simulink library "MCU_MAIN_LIB"  (R2023b)
settings: Solver=VariableStepAuto  StartTime=0.0  StopTime=10.0  RelTol=1e-3
undefined symbols (not defined in the file): BMS_MAIN_LIB, Error_Set_Reset_Deb_100MS, SAMPLE_TIME_100MS, SAMPLE_TIME_100MS_f32, SAMPLE_TIME_10MS
libraries: $bdroot x2, simulink x1
settings Model: Creator=Somashekar M  LastModifiedBy=Somashekar M

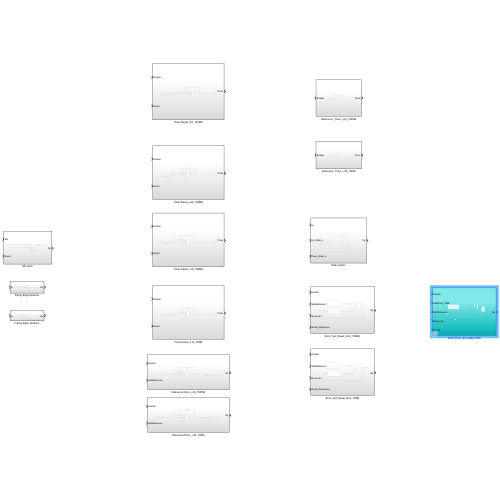
[thumbnail: Simulink's stored preview of the top-level diagram]
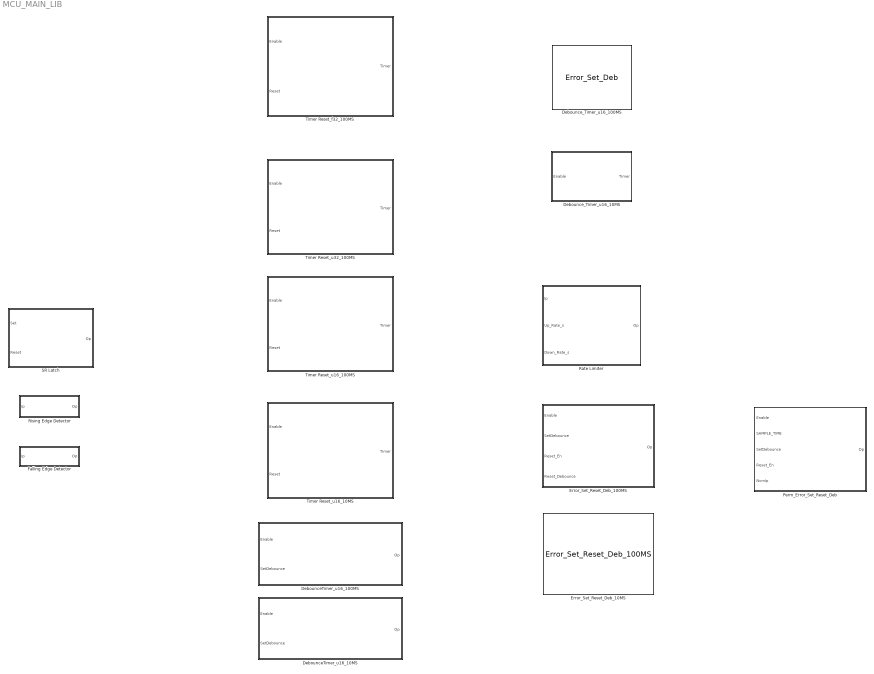
== system MCU_MAIN_LIB ==
  DebounceTimer_u16_100MS : Subsystem
  DebounceTimer_u16_10MS : Subsystem
  Debounce_Timer_u16_100MS : $bdroot/Error_Set_Reset_Deb_100MS/Error_Set_Deb  SystemSampleTime=-1  VariantActivationTime=update diagram  AllowFlexibleInterface=on  Latency=0  AutoFrameSizeCalculation=off
  Debounce_Timer_u16_10MS : Subsystem
  Error_Set_Reset_Deb_100MS : Subsystem
  Error_Set_Reset_Deb_10MS : $bdroot/Error_Set_Reset_Deb_100MS  SystemSampleTime=-1  VariantActivationTime=update diagram  AllowFlexibleInterface=on  Latency=0  AutoFrameSizeCalculation=off
      link override Error_Reset_Deb/Constant7: Value=SAMPLE_TIME_10MS
      link override Error_Set_Deb/Constant7: Value=SAMPLE_TIME_10MS
  Falling Edge Detector : Subsystem
  Perm_Error_Set_Reset_Deb : Subsystem  AncestorBlock=BMS_MAIN_LIB/Error_Set_Reset_Deb_100MS
  Rate Limiter : Subsystem
  Rising Edge Detector : Subsystem
  SR Latch : Subsystem
  Timer Reset_f32_100MS : Subsystem
  Timer Reset_u16_100MS : Subsystem
  Timer Reset_u16_10MS : Subsystem
  Timer Reset_u32_100MS : Subsystem

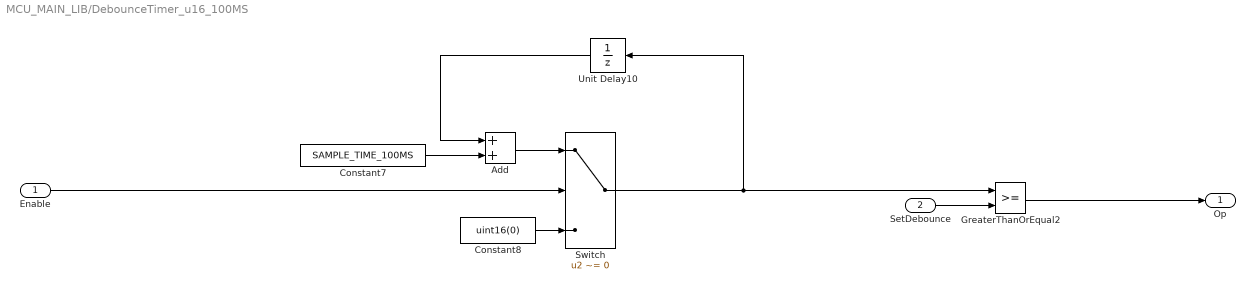
== system MCU_MAIN_LIB/DebounceTimer_u16_100MS ==
  Enable : Inport
  SetDebounce : Inport  Port=2
  Add : Sum
  Constant7 : Constant  Value=SAMPLE_TIME_100MS
  Constant8 : Constant  Value=uint16(0)
  GreaterThanOrEqual2 : RelationalOperator  OutDataTypeStr=boolean  RndMeth=Simplest  InputSameDT=off
  Switch : Switch  Criteria=u2 ~= 0  SaturateOnIntegerOverflow=off  InputSameDT=off
  Unit Delay10 : UnitDelay  SampleTime=-1  HasFrameUpgradeWarning=on
  Op : Outport
  wires:
  Add/1 -> Switch/1
  Constant7/1 -> Add/2
  Enable/1 -> Switch/2
  Unit Delay10/1 -> Add/1
  Constant8/1 -> Switch/3
  Switch/1 -> GreaterThanOrEqual2/1, Unit Delay10/1
  SetDebounce/1 -> GreaterThanOrEqual2/2
  GreaterThanOrEqual2/1 -> Op/1

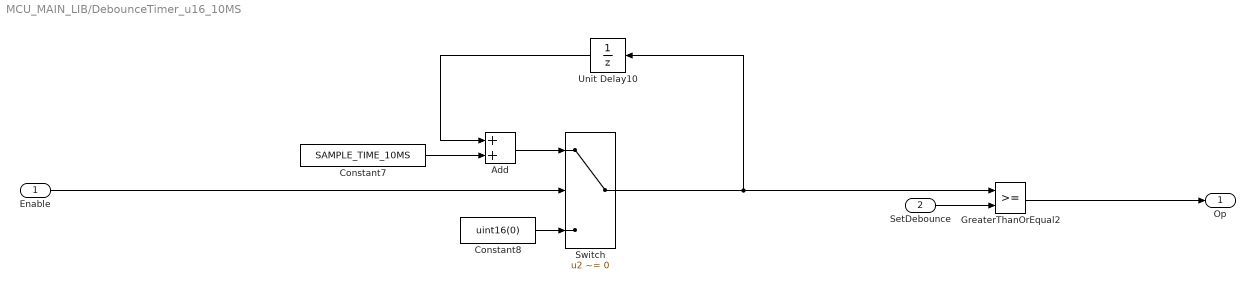
== system MCU_MAIN_LIB/DebounceTimer_u16_10MS ==
  Enable : Inport
  SetDebounce : Inport  Port=2
  Add : Sum
  Constant7 : Constant  Value=SAMPLE_TIME_10MS
  Constant8 : Constant  Value=uint16(0)
  GreaterThanOrEqual2 : RelationalOperator  OutDataTypeStr=boolean  RndMeth=Simplest  InputSameDT=off
  Switch : Switch  Criteria=u2 ~= 0  SaturateOnIntegerOverflow=off  InputSameDT=off
  Unit Delay10 : UnitDelay  SampleTime=-1  HasFrameUpgradeWarning=on
  Op : Outport
  wires:
  GreaterThanOrEqual2/1 -> Op/1
  SetDebounce/1 -> GreaterThanOrEqual2/2
  Switch/1 -> Unit Delay10/1, GreaterThanOrEqual2/1
  Constant8/1 -> Switch/3
  Unit Delay10/1 -> Add/1
  Enable/1 -> Switch/2
  Constant7/1 -> Add/2
  Add/1 -> Switch/1

== system MCU_MAIN_LIB/Debounce_Timer_u16_10MS ==
  Enable : Inport
  Add1 : Sum
  Constant7 : Constant  Value=SAMPLE_TIME_10MS
  Constant8 : Constant  Value=uint16(0)
  Switch2 : Switch  Criteria=u2 ~= 0  SaturateOnIntegerOverflow=off  InputSameDT=off
  Unit Delay10 : UnitDelay  SampleTime=-1  HasFrameUpgradeWarning=on
  Timer : Outport
  wires:
  Switch2/1 -> Timer/1, Unit Delay10/1
  Add1/1 -> Switch2/1
  Constant8/1 -> Switch2/3
  Enable/1 -> Switch2/2
  Unit Delay10/1 -> Add1/1
  Constant7/1 -> Add1/2

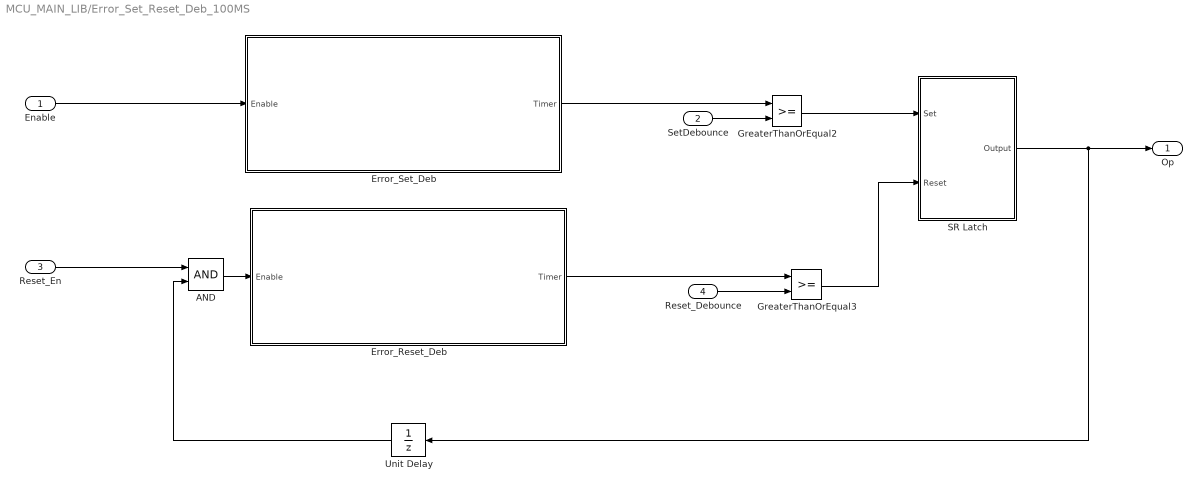
== system MCU_MAIN_LIB/Error_Set_Reset_Deb_100MS ==
  Enable : Inport
  SetDebounce : Inport  Port=2
  Reset_En : Inport  Port=3
  Reset_Debounce : Inport  Port=4
  AND : Logic  AllPortsSameDT=off  OutDataTypeStr=boolean
  Error_Reset_Deb : Subsystem
  Error_Set_Deb : Subsystem
  GreaterThanOrEqual2 : RelationalOperator  OutDataTypeStr=boolean  RndMeth=Simplest  InputSameDT=off
  GreaterThanOrEqual3 : RelationalOperator  OutDataTypeStr=boolean  RndMeth=Simplest  InputSameDT=off
  SR Latch : Subsystem
  Unit Delay : UnitDelay  SampleTime=-1  HasFrameUpgradeWarning=on
  Op : Outport
  wires:
  SetDebounce/1 -> GreaterThanOrEqual2/2
  Reset_Debounce/1 -> GreaterThanOrEqual3/2
  GreaterThanOrEqual3/1 -> SR Latch/2(Reset)
  GreaterThanOrEqual2/1 -> SR Latch/1(Set)
  SR Latch/1(Output) -> Op/1, Unit Delay/1
  AND/1 -> Error_Reset_Deb/1(Enable)
  Error_Set_Deb/1(Timer) -> GreaterThanOrEqual2/1
  Error_Reset_Deb/1(Timer) -> GreaterThanOrEqual3/1
  Reset_En/1 -> AND/1
  Unit Delay/1 -> AND/2
  Enable/1 -> Error_Set_Deb/1(Enable)

== system MCU_MAIN_LIB/Falling Edge Detector ==
  Ip : Inport
  AND : Logic  AllPortsSameDT=off  OutDataTypeStr=boolean
  NOT1 : Logic  Operator=NOT  IconShape=distinctive  AllPortsSameDT=off  OutDataTypeStr=boolean
  Unit Delay : UnitDelay  SampleTime=-1  HasFrameUpgradeWarning=on
  Op : Outport
  wires:
  Unit Delay/1 -> AND/2
  AND/1 -> Op/1
  Ip/1 -> NOT1/1, Unit Delay/1
  NOT1/1 -> AND/1

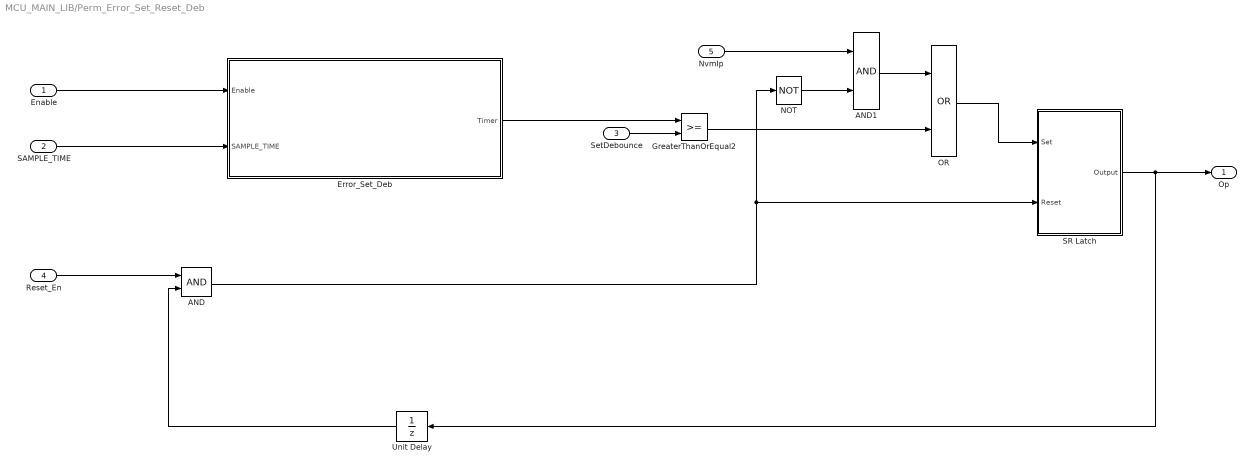
== system MCU_MAIN_LIB/Perm_Error_Set_Reset_Deb ==
  Enable : Inport
  SAMPLE_TIME : Inport  Port=2
  SetDebounce : Inport  Port=3
  Reset_En : Inport  Port=4
  NvmIp : Inport  Port=5
  AND : Logic  AllPortsSameDT=off  OutDataTypeStr=boolean
  AND1 : Logic  AllPortsSameDT=off  OutDataTypeStr=boolean
  Error_Set_Deb : Subsystem
  GreaterThanOrEqual2 : RelationalOperator  OutDataTypeStr=boolean  RndMeth=Simplest  InputSameDT=off
  NOT : Logic  Operator=NOT  IconShape=distinctive  AllPortsSameDT=off  OutDataTypeStr=boolean
  OR : Logic  Operator=OR  AllPortsSameDT=off  OutDataTypeStr=boolean
  SR Latch : Subsystem
  Unit Delay : UnitDelay  SampleTime=-1  HasFrameUpgradeWarning=on
  Op : Outport
  wires:
  Enable/1 -> Error_Set_Deb/1(Enable)
  Unit Delay/1 -> AND/2
  Reset_En/1 -> AND/1
  Error_Set_Deb/1(Timer) -> GreaterThanOrEqual2/1
  SR Latch/1(Output) -> Unit Delay/1, Op/1
  GreaterThanOrEqual2/1 -> OR/2
  AND/1 -> SR Latch/2(Reset), NOT/1
  SetDebounce/1 -> GreaterThanOrEqual2/2
  SAMPLE_TIME/1 -> Error_Set_Deb/2(SAMPLE_TIME)
  OR/1 -> SR Latch/1(Set)
  AND1/1 -> OR/1
  NvmIp/1 -> AND1/1
  NOT/1 -> AND1/2

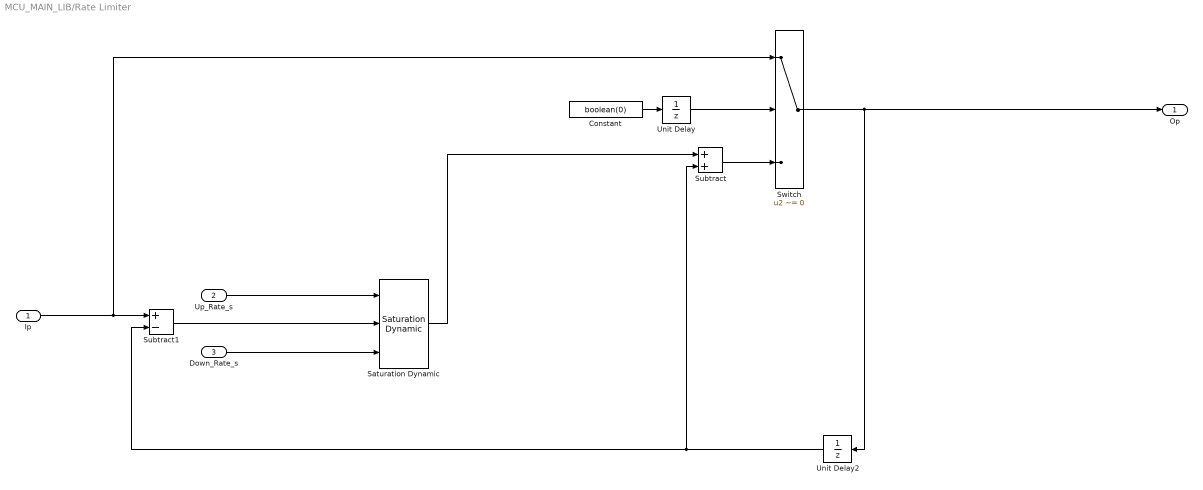
== system MCU_MAIN_LIB/Rate Limiter ==
  Ip : Inport
  Up_Rate_s : Inport  Port=2
  Down_Rate_s : Inport  Port=3
  Constant : Constant  Value=boolean(0)
  Saturation Dynamic : simulink/Discontinuities/Saturation Dynamic  OutMin=[]  OutMax=[]  OutDataTypeStr=Inherit: Same as second input  OutDataType=fixdt(1, 16)  OutScaling=2^-10  DoSatur=off
  Subtract : Sum
  Subtract1 : Sum  Inputs=+-
  Switch : Switch  Criteria=u2 ~= 0  SaturateOnIntegerOverflow=off  InputSameDT=off
  Unit Delay : UnitDelay  InitialCondition=boolean(1)  SampleTime=-1  HasFrameUpgradeWarning=on
  Unit Delay2 : UnitDelay  SampleTime=-1  HasFrameUpgradeWarning=on
  Op : Outport
  wires:
  Subtract/1 -> Switch/3
  Unit Delay/1 -> Switch/2
  Constant/1 -> Unit Delay/1
  Ip/1 -> Switch/1, Subtract1/1
  Down_Rate_s/1 -> Saturation Dynamic/3
  Unit Delay2/1 -> Subtract/2, Subtract1/2
  Subtract1/1 -> Saturation Dynamic/2
  Saturation Dynamic/1 -> Subtract/1
  Switch/1 -> Op/1, Unit Delay2/1
  Up_Rate_s/1 -> Saturation Dynamic/1

== system MCU_MAIN_LIB/Rising Edge Detector ==
  Ip : Inport
  AND : Logic  AllPortsSameDT=off  OutDataTypeStr=boolean
  NOT : Logic  Operator=NOT  IconShape=distinctive  AllPortsSameDT=off  OutDataTypeStr=boolean
  Unit Delay : UnitDelay  SampleTime=-1  HasFrameUpgradeWarning=on
  Op : Outport
  wires:
  Ip/1 -> Unit Delay/1, AND/1
  AND/1 -> Op/1
  NOT/1 -> AND/2
  Unit Delay/1 -> NOT/1

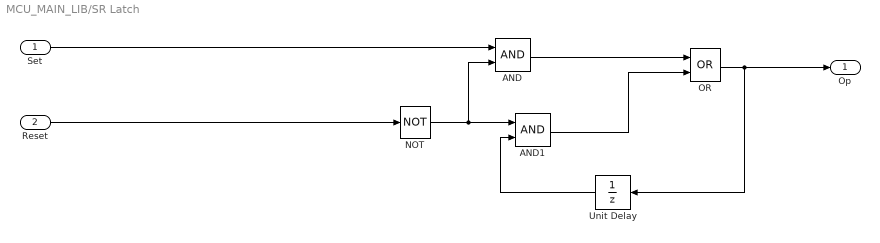
== system MCU_MAIN_LIB/SR Latch ==
  Set : Inport
  Reset : Inport  Port=2
  AND : Logic  AllPortsSameDT=off  OutDataTypeStr=boolean
  AND1 : Logic  AllPortsSameDT=off  OutDataTypeStr=boolean
  NOT : Logic  Operator=NOT  IconShape=distinctive  AllPortsSameDT=off  OutDataTypeStr=boolean
  OR : Logic  Operator=OR  AllPortsSameDT=off  OutDataTypeStr=boolean
  Unit Delay : UnitDelay  SampleTime=-1  HasFrameUpgradeWarning=on
  Op : Outport
  wires:
  Unit Delay/1 -> AND1/2
  Set/1 -> AND/1
  AND1/1 -> OR/2
  NOT/1 -> AND1/1, AND/2
  OR/1 -> Unit Delay/1, Op/1
  AND/1 -> OR/1
  Reset/1 -> NOT/1

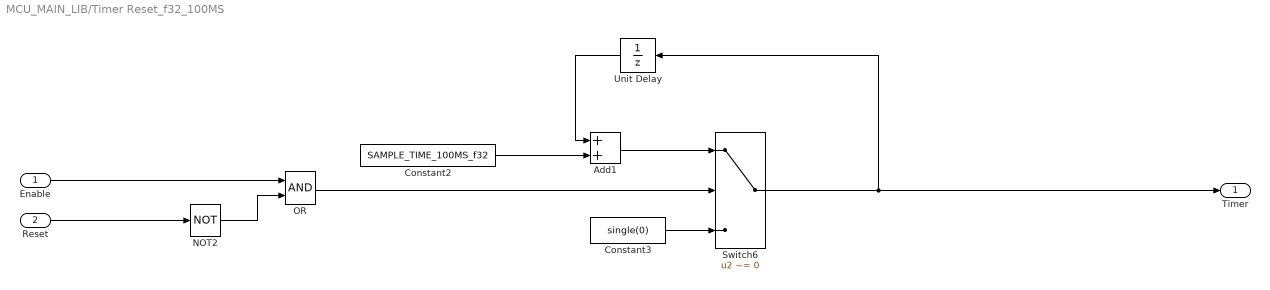
== system MCU_MAIN_LIB/Timer Reset_f32_100MS ==
  Enable : Inport
  Reset : Inport  Port=2
  Add1 : Sum
  Constant2 : Constant  Value=SAMPLE_TIME_100MS_f32  OutDataTypeStr=single
  Constant3 : Constant  Value=single(0)
  NOT2 : Logic  Operator=NOT  IconShape=distinctive  AllPortsSameDT=off  OutDataTypeStr=boolean
  OR : Logic  AllPortsSameDT=off  OutDataTypeStr=boolean
  Switch6 : Switch  Criteria=u2 ~= 0  SaturateOnIntegerOverflow=off  InputSameDT=off
  Unit Delay : UnitDelay  SampleTime=-1  HasFrameUpgradeWarning=on
  Timer : Outport
  wires:
  Enable/1 -> OR/1
  Constant3/1 -> Switch6/3
  Add1/1 -> Switch6/1
  Switch6/1 -> Timer/1, Unit Delay/1
  Reset/1 -> NOT2/1
  NOT2/1 -> OR/2
  OR/1 -> Switch6/2
  Unit Delay/1 -> Add1/1
  Constant2/1 -> Add1/2

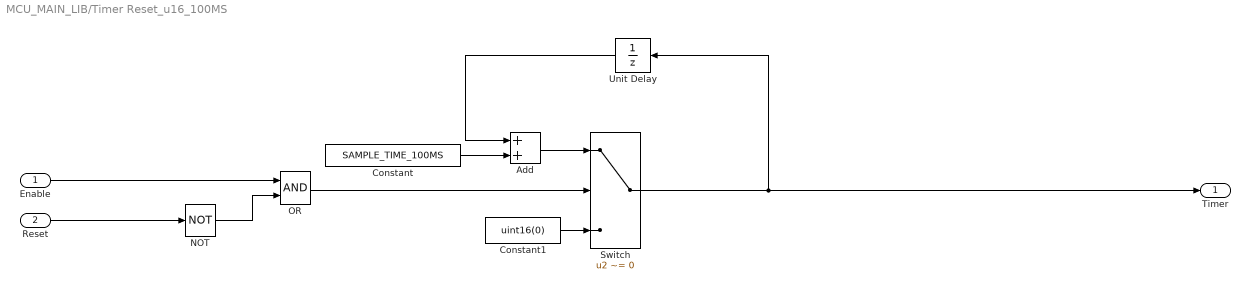
== system MCU_MAIN_LIB/Timer Reset_u16_100MS ==
  Enable : Inport
  Reset : Inport  Port=2
  Add : Sum
  Constant : Constant  Value=SAMPLE_TIME_100MS  OutDataTypeStr=uint16
  Constant1 : Constant  Value=uint16(0)
  NOT : Logic  Operator=NOT  IconShape=distinctive  AllPortsSameDT=off  OutDataTypeStr=boolean
  OR : Logic  AllPortsSameDT=off  OutDataTypeStr=boolean
  Switch : Switch  Criteria=u2 ~= 0  SaturateOnIntegerOverflow=off  InputSameDT=off
  Unit Delay : UnitDelay  SampleTime=-1  HasFrameUpgradeWarning=on
  Timer : Outport
  wires:
  Enable/1 -> OR/1
  Switch/1 -> Timer/1, Unit Delay/1
  Unit Delay/1 -> Add/1
  Constant/1 -> Add/2
  Add/1 -> Switch/1
  Constant1/1 -> Switch/3
  Reset/1 -> NOT/1
  NOT/1 -> OR/2
  OR/1 -> Switch/2

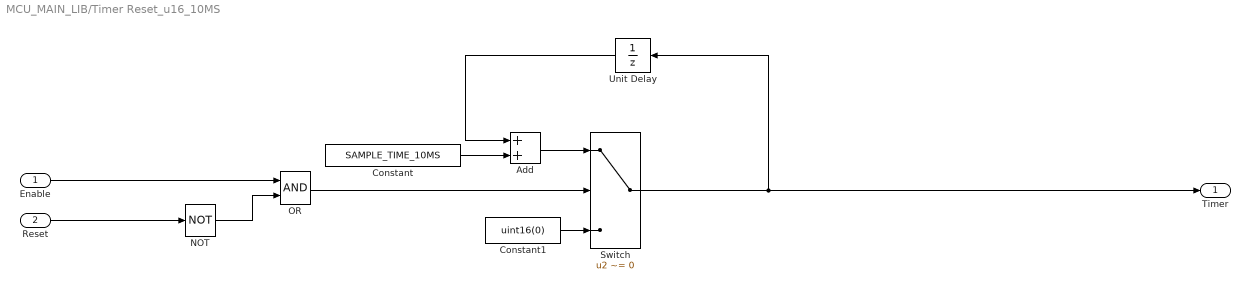
== system MCU_MAIN_LIB/Timer Reset_u16_10MS ==
  Enable : Inport
  Reset : Inport  Port=2
  Add : Sum
  Constant : Constant  Value=SAMPLE_TIME_10MS  OutDataTypeStr=uint16
  Constant1 : Constant  Value=uint16(0)
  NOT : Logic  Operator=NOT  IconShape=distinctive  AllPortsSameDT=off  OutDataTypeStr=boolean
  OR : Logic  AllPortsSameDT=off  OutDataTypeStr=boolean
  Switch : Switch  Criteria=u2 ~= 0  SaturateOnIntegerOverflow=off  InputSameDT=off
  Unit Delay : UnitDelay  SampleTime=-1  HasFrameUpgradeWarning=on
  Timer : Outport
  wires:
  OR/1 -> Switch/2
  NOT/1 -> OR/2
  Reset/1 -> NOT/1
  Constant1/1 -> Switch/3
  Add/1 -> Switch/1
  Constant/1 -> Add/2
  Unit Delay/1 -> Add/1
  Switch/1 -> Unit Delay/1, Timer/1
  Enable/1 -> OR/1

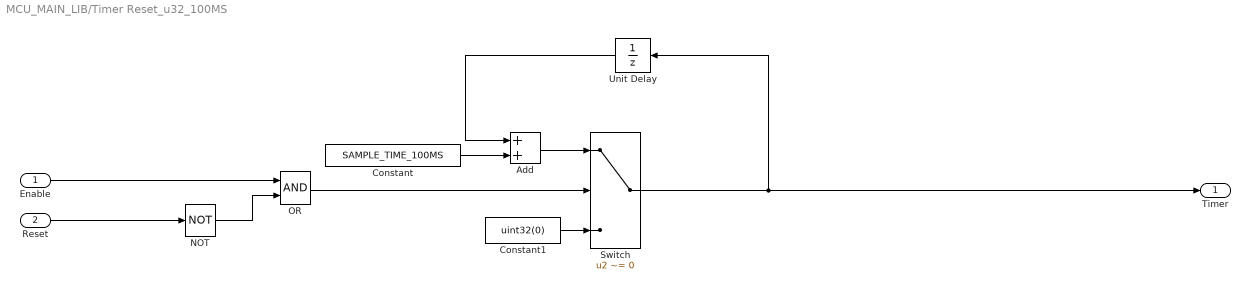
== system MCU_MAIN_LIB/Timer Reset_u32_100MS ==
  Enable : Inport
  Reset : Inport  Port=2
  Add : Sum
  Constant : Constant  Value=SAMPLE_TIME_100MS  OutDataTypeStr=uint32
  Constant1 : Constant  Value=uint32(0)
  NOT : Logic  Operator=NOT  IconShape=distinctive  AllPortsSameDT=off  OutDataTypeStr=boolean
  OR : Logic  AllPortsSameDT=off  OutDataTypeStr=boolean
  Switch : Switch  Criteria=u2 ~= 0  SaturateOnIntegerOverflow=off  InputSameDT=off
  Unit Delay : UnitDelay  SampleTime=-1  HasFrameUpgradeWarning=on
  Timer : Outport
  wires:
  OR/1 -> Switch/2
  NOT/1 -> OR/2
  Reset/1 -> NOT/1
  Constant1/1 -> Switch/3
  Add/1 -> Switch/1
  Constant/1 -> Add/2
  Unit Delay/1 -> Add/1
  Switch/1 -> Unit Delay/1, Timer/1
  Enable/1 -> OR/1

== system MCU_MAIN_LIB/Error_Set_Reset_Deb_100MS/Error_Reset_Deb ==
  Enable : Inport
  Add : Sum
  Constant7 : Constant  Value=SAMPLE_TIME_100MS
  Constant8 : Constant  Value=uint16(0)
  Switch : Switch  Criteria=u2 ~= 0  SaturateOnIntegerOverflow=off  InputSameDT=off
  Unit Delay10 : UnitDelay  SampleTime=-1  HasFrameUpgradeWarning=on
  Timer : Outport
  wires:
  Switch/1 -> Unit Delay10/1, Timer/1
  Constant8/1 -> Switch/3
  Unit Delay10/1 -> Add/1
  Enable/1 -> Switch/2
  Constant7/1 -> Add/2
  Add/1 -> Switch/1

== system MCU_MAIN_LIB/Error_Set_Reset_Deb_100MS/Error_Set_Deb ==
  Enable : Inport
  Add : Sum
  Constant7 : Constant  Value=SAMPLE_TIME_100MS
  Constant8 : Constant  Value=uint16(0)
  Switch : Switch  Criteria=u2 ~= 0  SaturateOnIntegerOverflow=off  InputSameDT=off
  Unit Delay10 : UnitDelay  SampleTime=-1  HasFrameUpgradeWarning=on
  Timer : Outport
  wires:
  Add/1 -> Switch/1
  Constant7/1 -> Add/2
  Enable/1 -> Switch/2
  Unit Delay10/1 -> Add/1
  Constant8/1 -> Switch/3
  Switch/1 -> Timer/1, Unit Delay10/1

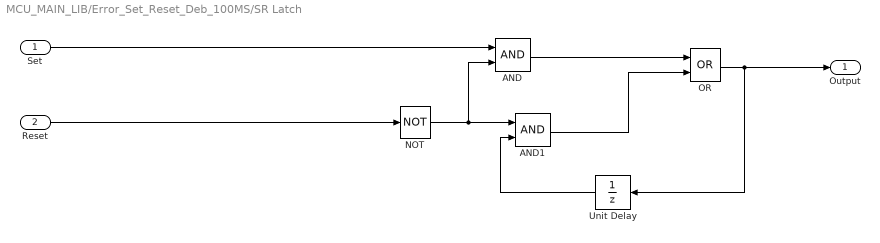
== system MCU_MAIN_LIB/Error_Set_Reset_Deb_100MS/SR Latch ==
  Set : Inport
  Reset : Inport  Port=2
  AND : Logic  AllPortsSameDT=off  OutDataTypeStr=boolean
  AND1 : Logic  AllPortsSameDT=off  OutDataTypeStr=boolean
  NOT : Logic  Operator=NOT  IconShape=distinctive  AllPortsSameDT=off  OutDataTypeStr=boolean
  OR : Logic  Operator=OR  AllPortsSameDT=off  OutDataTypeStr=boolean
  Unit Delay : UnitDelay  SampleTime=-1  HasFrameUpgradeWarning=on
  Output : Outport
  wires:
  Unit Delay/1 -> AND1/2
  Set/1 -> AND/1
  AND1/1 -> OR/2
  NOT/1 -> AND1/1, AND/2
  OR/1 -> Unit Delay/1, Output/1
  AND/1 -> OR/1
  Reset/1 -> NOT/1

== system MCU_MAIN_LIB/Perm_Error_Set_Reset_Deb/Error_Set_Deb ==
  Enable : Inport
  SAMPLE_TIME : Inport  Port=2
  Add : Sum
  Constant8 : Constant  Value=uint16(0)
  Switch : Switch  Criteria=u2 ~= 0  SaturateOnIntegerOverflow=off  InputSameDT=off
  Unit Delay10 : UnitDelay  SampleTime=-1  HasFrameUpgradeWarning=on
  Timer : Outport
  wires:
  Switch/1 -> Unit Delay10/1, Timer/1
  Constant8/1 -> Switch/3
  Unit Delay10/1 -> Add/1
  Enable/1 -> Switch/2
  SAMPLE_TIME/1 -> Add/2
  Add/1 -> Switch/1

== system MCU_MAIN_LIB/Perm_Error_Set_Reset_Deb/SR Latch ==
  Set : Inport
  Reset : Inport  Port=2
  AND : Logic  AllPortsSameDT=off  OutDataTypeStr=boolean
  AND1 : Logic  AllPortsSameDT=off  OutDataTypeStr=boolean
  NOT : Logic  Operator=NOT  IconShape=distinctive  AllPortsSameDT=off  OutDataTypeStr=boolean
  OR : Logic  Operator=OR  AllPortsSameDT=off  OutDataTypeStr=boolean
  Unit Delay : UnitDelay  SampleTime=-1  HasFrameUpgradeWarning=on
  Output : Outport
  wires:
  Reset/1 -> NOT/1
  AND/1 -> OR/1
  OR/1 -> Output/1, Unit Delay/1
  NOT/1 -> AND/2, AND1/1
  AND1/1 -> OR/2
  Set/1 -> AND/1
  Unit Delay/1 -> AND1/2
